simulink model "Node_NM"  (R2024b)
settings: Solver=ode1  StartTime=0.0  StopTime=10.0  FixedStep=0.5e-3  RelTol=1e-3
values from neighbouring files (symbols this model uses):
  zero_path_cfg = 1.0    [NM_dd.sldd]
settings Model: DataDictionary=NM_dd.sldd  EnableAccessToBaseWorkspace=off  NumberOfSteps=100  Creator=wai484  LastModifiedBy=wai484
settings SolverCC: EnableFixedStepZeroCrossing=on
settings DataIOCC: SaveOutput=off  SignalLogging=off  DSMLogging=off  SaveTime=off  ReturnWorkspaceOutputs=off
settings OptimizationCC: SimCompilerOptimization=on
settings DebuggingCC: SignalInfNanChecking=error  CheckMatrixSingularityMsg=warning
settings ModelReferenceCC: EnableParallelModelReferenceBuilds=on  ModelReferenceMinAlgLoopOccurrences=on
settings RTWCC: BuildConfiguration=Faster Runs
settings GRTTargetCC: CombineOutputUpdateFcns=off  OptimizeReductions=on

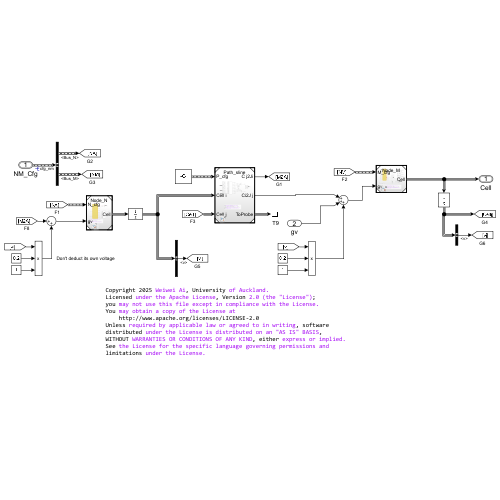
[thumbnail: Simulink's stored preview of the top-level diagram]
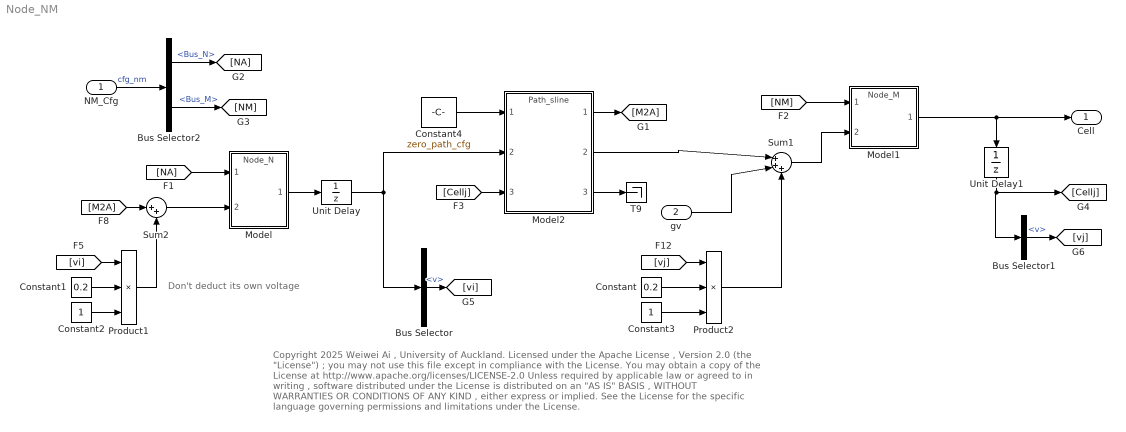
== system Node_NM ==
  note: Don't deduct its own voltage
  note: Copyright 2025 Weiwei Ai , University of Auckland.
      | Licensed under the Apache License , Version 2.0 (the "License") ;
      | you may not use this file except in compliance with the License.
      | You may obtain a copy of the License at
      | http://www.apache.org/licenses/LICENSE-2.0
      | Unless required by applicable law or agreed to in writing , software
      | distributed under the License is distributed on an "AS IS" BASIS ,
      | WITHOUT WARRANTIES OR CONDITIONS OF ANY KIND , either express or implied.
      | See the License for the specific language governing permissions and
      | limitations under the License.
  NM_Cfg : Inport  OutDataTypeStr=Bus: Config_NM  BusOutputAsStruct=on
  gv : Inport  Port=2  OutDataTypeStr=double  PortDimensions=1
  Bus Selector : BusSelector  OutputSignals=v
  Bus Selector1 : BusSelector  OutputSignals=v
  Bus Selector2 : BusSelector  OutputSignals=Bus_N,Bus_M
  Constant : Constant  Value=0.2
  Constant1 : Constant  Value=0.2
  Constant2 : Constant
  Constant3 : Constant
  Constant4 : Constant  Value=zero_path_cfg  VectorParams1D=off  OutDataTypeStr=Bus: Config_Path  SampleTime=-1
  Model : ModelReference  ModelNameDialog=Node_N.slx  SimulationMode=Normal  ModelReferenceVersion=1.94
  Model1 : ModelReference  ModelNameDialog=Node_M.slx  SimulationMode=Normal  ModelReferenceVersion=1.73
  Model2 : ModelReference  ModelNameDialog=Path_sline.slx  UsingDefaultArgumentValue=0,0,0,0,0,0  SimulationMode=Normal  ModelReferenceVersion=1.55
  Product1 : Product  Inputs=***
  Product2 : Product  Inputs=***
  Sum1 : Sum  Inputs=|+++
  Sum2 : Sum  Inputs=|++
  T9 : Terminator
  Unit Delay : UnitDelay  SampleTime=-1  HasFrameUpgradeWarning=on
  Unit Delay1 : UnitDelay  SampleTime=-1  HasFrameUpgradeWarning=on
  Cell : Outport  OutDataTypeStr=Bus: Cell  SampleTime=0
  wires:
  Model2/3 -> T9/1
  [NA] -> Model/1
  [NM] -> Model1/1
  [Cellj] -> Model2/3
  Model/1 -> Unit Delay/1
  Constant/1 -> Product2/2
  [vj] -> Product2/1
  Product2/1 -> Sum1/3
  [M2A] -> Sum2/1
  Constant1/1 -> Product1/2
  [vi] -> Product1/1
  Product1/1 -> Sum2/2
  Constant3/1 -> Product2/3
  gv/1 -> Sum1/2
  Constant2/1 -> Product1/3
  Bus Selector/1 -> [vi]  "<v>"
  Bus Selector1/1 -> [vj]  "<v>"
  Constant4/1 -> Model2/1
  NM_Cfg/1 -> Bus Selector2/1  "cfg_nm"
  Bus Selector2/1 -> [NA]  "<Bus_N>"
  Bus Selector2/2 -> [NM]  "<Bus_M>"
  Model2/2 -> Sum1/1
  Model2/1 -> [M2A]
  Unit Delay/1 -> Bus Selector/1, Model2/2
  Model1/1 -> Unit Delay1/1, Cell/1
  Sum1/1 -> Model1/2
  Sum2/1 -> Model/2
  Unit Delay1/1 -> Bus Selector1/1, [Cellj]
